simulink model "test_cosim_hydraulics"  (Simulink 7.4)
settings: Solver=ode15s  StartTime=0.0  StopTime=20.0  MaxStep=0.2  RelTol=1e-3
InitFcn:
  | valve_orifice_area = 0.16;
  | x0 = 0.8;
undefined symbols (not defined in the file): CEcosimulation, CoSimulate1, sigbuilder_block
libraries: fl_lib x21, sh_lib x10, nesl_utility x9, instrumentlib x2
Description:
  | Power-Assisted Steering Mechanism
  | 
  | The model represents a simplified version of a power-assisted steering mechanism
  | showing all its major parts: double-acting hydraulic cylinder; rotational valve; fixed-
  | displacement pump;  pressure-relief valve; mechanical load consisting of a reduced
  | to a driving shaft inertia, damping, and stiffness; and torsion bar installed between the
  | steering wheel and the pinion of a rack-and-pinion mechanism.
  | The rotation of the steering wheel causes the torsion bar to twist with respect to the
  | pinion position. The deformation of the bar is transformed into opening of the rotational
  | valve, which connects ports of the cylinder to pressure or exhaust lines depending on
  | the direction of rotation. If deformation exceeds 9 deg the wheel is connected directly
  | to the pinion through the hard stops installed in parallel with the torsion bar.
  | The cylinder moves the steering rods and, at the same time, twists the torsion rod
  | in the opposite direction until the valve is in neutral position.
  | 
  | 
  | Copyright 2008-2009 The MathWorks(TM), Inc.
settings Model: Creator=vtchkalo  LastModifiedBy=tasora  ExtModeAutoUpdateStatusClock=off
settings SolverCC: InitialStep=1e-6
settings OptimizationCC: InitFltsAndDblsToZero=on
settings DebuggingCC: SaveWithParameterizedLinksMsg=none  SignalResolutionControl=TryResolveAllWithWarning  SolverPrmCheckMsg=none
settings GRTTargetCC: TargetFcnLib=ansi_tfl_tmw.mat

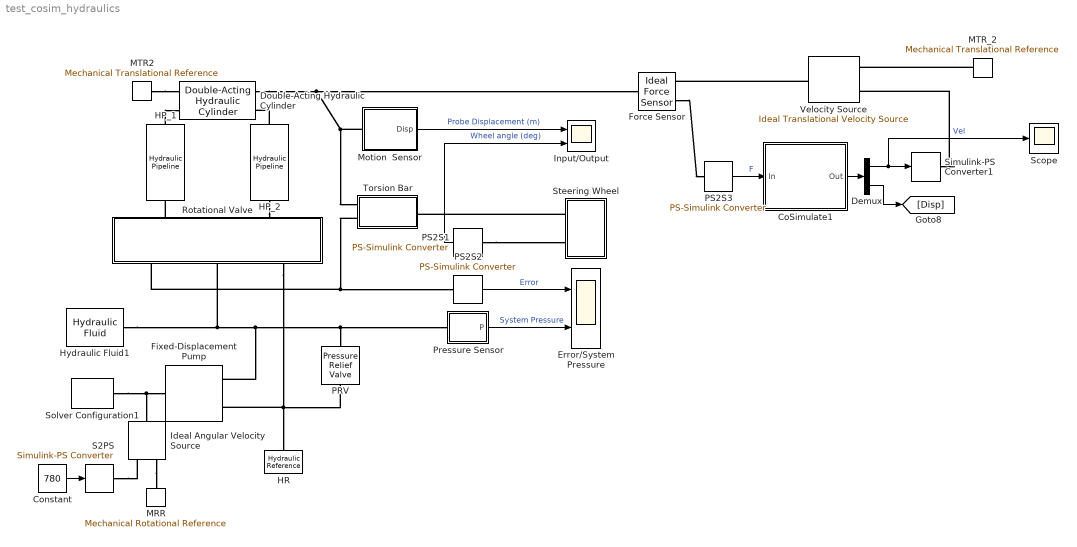
== system test_cosim_hydraulics ==
  CoSimulate1 : Subsystem  Description=|  Priority=100  AncestorBlock=CEcosimulation/CoSimulate1  mask{com_step=0.001, tcp_data_size=2, host_name=localhost, tcp_port=50009, tcp_timeout=15}
      | This block can be used to exchange data with Chrono::Engine.                                                                                      
      | A Chrono::Engine program with a running ChCosimulation inferface must be started, it will work as a server; then the Simulink program must be run.
      | Note! check that the dimensions of the exchanged vectors do match!
      mask prompts: com_step "Communication step size"; tcp_data_size "N. of scalars received from C::E (as block output)"; host_name "TCP host name (ex. 'localhost', or 'www.myhost.com')"; tcp_port "TCP port (ex. 50007)"; tcp_timeout "TCP timeout (seconds)"
      mask init:
      | block_receive = [gcb, '/TCP Receive'];
      | set_param(block_receive, 'SampleTime', num2str(com_step));
      | set_param(block_receive, 'Host', host_name);
      | set_param(block_receive, 'Port', num2str(tcp_port));
      | set_param(block_receive, 'DataSize', num2str(tcp_data_size+1));
      | set_param(block_receive, 'Timeout', num2str(tcp_timeout));
      | block_send = [gcb, '/TCP Send'];
      | set_param(block_send, 'Host', host_name);
      | set_param(block_send, 'Port', num2str(tcp_port));
      mask Display:
      | image(imread('block_logo.png'))
      | disp('C::E                   ')
  Constant : Constant  Value=780  OutDataType=sfix(16)  OutScaling=2^0
  Demux : Demux  Outputs=2
  Double-Acting Hydraulic Cylinder : sh_lib/Hydraulic Cylinders/Double-Acting Hydraulic Cylinder  Tag=Factory Generic  DialogController=NetworkEngine.DynNeDlgSource  SystemSampleTime=-1  area_A=9.1 cm^2  area_B=9.1 cm^2  stroke=18.4 cm  init_pos=9.2 cm  dead_vol_A=1e-04 m^3  dead_vol_B=1e-04 m^3  k_sh=1.4  stiff=1e+06 N/m  D=150 N/(m/s)  or=1  LocalVarLogging=[]
  Error/System Pressure : Scope  NumInputPorts=2
      settings: TimeRange=20  YMin=-0.4~7  YMax=0.4~10  SaveName=ScopeDataCE
  Fixed-Displacement Pump : sh_lib/Pumps and Motors/Fixed-Displacement Pump  Tag=Factory Generic  DialogController=NetworkEngine.DynNeDlgSource  SystemSampleTime=-1  D=1.14e-06 m^3/rad  efficiency_vol=0.92  efficiency_tot=0.8  pr_nominal=1e+07 Pa  w_nominal=188 rad/s  visc_nominal=18 cSt  pump_delivery_Log=off  leakage_flow_Log=off  torque_Log=off  power_hyd_Log=off  pressure_diff_Log=off  shaft_ang_vel_Log=off  LocalVarNames=|pump_delivery|leakage_flow|torque|power_hyd|pressure_diff|shaft_ang_vel  LocalVarDescs=|Pump delivery (m^3/s)|Leakage flow rate (m^3/s)|Driving shaft torque (N*m)|Output flow power (W)|Pressure differential (Pa)|Driving shaft angular velocity (rad/s)  LocalVarLogging=[0 0 0 0 0 0]
  Force Sensor : fl_lib/Mechanical/Mechanical Sensors/Ideal Force Sensor  Tag=Factory Generic  DialogController=NetworkEngine.DynNeDlgSource  SystemSampleTime=-1  v_Log=off  f_Log=off  LocalVarNames=|v|f  LocalVarDescs=|v|f  LocalVarLogging=[]
  HP_1 : sh_lib/Pipelines/Hydraulic Pipeline  Tag=Factory Generic  DialogController=NetworkEngine.DynNeDlgSource  SystemSampleTime=-1  cs_type=1  d_in=6 mm  area=1e-04 m^2  D_h=0.0112 m  s_factor=64  length=1.8 m  length_ad=1 m  roughness=1.5e-05 m  Re_lam=2e+03  Re_turb=4e+03  wall_type=1  pr_r_coef=2e-12 m/Pa  time_const=0.01 s  k_sh=1.4  LocalVarLogging=[]
  HP_2 : sh_lib/Pipelines/Hydraulic Pipeline  Tag=Factory Generic  DialogController=NetworkEngine.DynNeDlgSource  SystemSampleTime=-1  cs_type=1  d_in=6 mm  area=1e-04 m^2  D_h=0.0112 m  s_factor=64  length=1.6 m  length_ad=1 m  roughness=1.5e-05 m  Re_lam=2e+03  Re_turb=4e+03  wall_type=1  pr_r_coef=2e-12 m/Pa  time_const=0.01 s  k_sh=1.4  LocalVarLogging=[]
  HR : fl_lib/Hydraulic/Hydraulic Elements/Hydraulic Reference  Tag=Factory Generic  DialogController=NetworkEngine.DynNeDlgSource  SystemSampleTime=-1  q_Log=off  LocalVarNames=|q  LocalVarDescs=|q  LocalVarLogging=[]
  Hydraulic Fluid1 : sh_lib/Hydraulic Utilities/Hydraulic Fluid  Tag=Factory Generic  DialogController=NetworkEngine.DynNeDlgSource  SystemSampleTime=-1  DataSource=1  SelFluid=9  SysTemp=60 c  TrapAir=0.005  ViscDerFactor=1  LocalVarLogging=[]
  Ideal Angular Velocity Source : fl_lib/Mechanical/Mechanical Sources/Ideal Angular Velocity Source  Tag=Factory Generic  DialogController=NetworkEngine.DynNeDlgSource  SystemSampleTime=-1  w_Log=off  t_Log=off  LocalVarNames=|torque|rel_velocity|power  LocalVarDescs=|Torque (N*m)|Relative velocity (rad/s)|Power generated by the sourcec(W)  LocalVarLogging=[0 0 0]
  Input/Output : Scope  NumInputPorts=2
      settings: TimeRange=20  YMin=-0.001~0  YMax=0.009~15
  MRR : fl_lib/Mechanical/Rotational Elements/Mechanical Rotational Reference  Tag=Factory Generic  DialogController=NetworkEngine.DynNeDlgSource  SystemSampleTime=-1  t_Log=off  LocalVarNames=|t  LocalVarDescs=|t  LocalVarLogging=[]
  MTR2 : fl_lib/Mechanical/Translational Elements/Mechanical Translational Reference  Tag=Factory Generic  DialogController=NetworkEngine.DynNeDlgSource  SystemSampleTime=-1  f_Log=off  LocalVarNames=|f  LocalVarDescs=|f  LocalVarLogging=[]
  MTR_2 : fl_lib/Mechanical/Translational Elements/Mechanical Translational Reference  Tag=Factory Generic  DialogController=NetworkEngine.DynNeDlgSource  SystemSampleTime=-1  f_Log=off  LocalVarNames=|f  LocalVarDescs=|f  LocalVarLogging=[]
  Motion  Sensor : Subsystem
  PRV : sh_lib/Valves/Pressure Control Valves/Pressure Relief Valve  Tag=Factory Generic  DialogController=NetworkEngine.DynNeDlgSource  SystemSampleTime=-1  area_max=0.46 cm^2  pres_set=12 bar  reg_range=2.1 bar  C_d=0.7  Re_cr=12  A_leak=1e-9 m^2  flow_rate_Log=off  pr_drop_Log=off  power_Log=off  area_Log=off  Re_Log=off  LocalVarNames=|flow_rate|pr_drop|power|area|Re  LocalVarDescs=|Flow rate through the valve (m^3/s)|Pressure differential across the valve (Pa)|Hydraulic loss power (W)|Instantaneous passage area (m^2)|Reynolds number  LocalVarLogging=[0 0 0 0 0]
  PS2S1 : nesl_utility/PS-Simulink Converter  DialogController=NetworkEngine.DynNeUtilDlgSource  SystemSampleTime=-1  PhysicalDomain=network_engine_domain  LeftPortType=input  RightPortType=output  SubClassName=ps_output  Unit=deg  AffineConversion=off
  PS2S2 : nesl_utility/PS-Simulink Converter  DialogController=NetworkEngine.DynNeUtilDlgSource  SystemSampleTime=-1  PhysicalDomain=network_engine_domain  LeftPortType=input  RightPortType=output  SubClassName=ps_output  Unit=deg  AffineConversion=off
  PS2S3 : nesl_utility/PS-Simulink Converter  DialogController=NetworkEngine.DynNeUtilDlgSource  SystemSampleTime=-1  PhysicalDomain=network_engine_domain  LeftPortType=input  RightPortType=output  SubClassName=ps_output  Unit=N  AffineConversion=off
  Pressure Sensor : Subsystem
  Rotational Valve : Subsystem
  S2PS : nesl_utility/Simulink-PS Converter  DialogController=NetworkEngine.DynNeUtilDlgSource  SystemSampleTime=-1  PhysicalDomain=network_engine_domain  LeftPortType=input  RightPortType=output  SubClassName=ps_input  Unit=rpm  AffineConversion=off  InputFilterTimeConstant=.001  UdotUserProvided=0
  Scope : Scope
  Simulink-PS Converter1 : nesl_utility/Simulink-PS Converter  DialogController=NetworkEngine.DynNeUtilDlgSource  SystemSampleTime=-1  PhysicalDomain=network_engine_domain  LeftPortType=input  RightPortType=output  SubClassName=ps_input  Unit=1  AffineConversion=off  InputFilterTimeConstant=.001  UdotUserProvided=0
  Solver Configuration1 : nesl_utility/Solver Configuration  DialogController=NetworkEngine.DynNeUtilDlgSource  SystemSampleTime=-1  PhysicalDomain=network_engine_domain  LeftPortType=input  RightPortType=generic  SubClassName=solver  Accelerate=off  Profile=off  Reg=off  Der=off  ResidualTolerance=1e-9  MaxNonlinIter=12  MaxModeIter=2  DoFixedCost=off  DoDC=off  LinearAlgebra=Sparse  LocalSolverSampleTime=.001  LocalSolverChoice=NE_BACKWARD_EULER_ADVANCER  UseLocalSolver=off
  Steering Wheel : Subsystem
  Torsion Bar : Subsystem
  Velocity Source : fl_lib/Mechanical/Mechanical Sources/Ideal Translational Velocity Source  DialogController=NetworkEngine.DynNeDlgSource  SystemSampleTime=-1  v_Log=off  f_Log=off  LocalVarNames=|v|f  LocalVarDescs=|v|f  LocalVarLogging=[0 0]
  wires:
  Constant/1 -> S2PS/1
  Motion  Sensor/1(Disp) -> Input/Output/1  "Probe Displacement (m)"
  PS2S1/1 -> Input/Output/2  "Wheel angle (deg)"
  PS2S2/1 -> Error/System Pressure/1  "Error"
  Pressure Sensor/1(P) -> Error/System Pressure/2  "System Pressure"
  PS2S3/1 -> CoSimulate1/1(In)  "F"
  CoSimulate1/1(Out) -> Demux/1
  Demux/1 -> Simulink-PS Converter1/1, Scope/1  "Vel"
  Demux/2 -> [Disp]
  connections:
  Double-Acting Hydraulic Cylinder/RConn1 -- Torsion Bar/RConn1 -- Motion  Sensor/LConn1 -- Force Sensor/LConn1
  HP_2/RConn1 -- Rotational Valve/RConn2
  Steering Wheel/RConn1 -- Torsion Bar/LConn1
  Rotational Valve/RConn1 -- HP_1/LConn1
  HP_1/RConn1 -- Double-Acting Hydraulic Cylinder/LConn2
  Ideal Angular Velocity Source/RConn2 -- MRR/LConn1
  MTR2/LConn1 -- Double-Acting Hydraulic Cylinder/LConn1
  HP_2/LConn1 -- Double-Acting Hydraulic Cylinder/RConn2
  S2PS/RConn1 -- Ideal Angular Velocity Source/RConn1
  Solver Configuration1/RConn1 -- Fixed-Displacement Pump/LConn1 -- Ideal Angular Velocity Source/LConn1
  PS2S1/LConn1 -- Steering Wheel/RConn2
  Torsion Bar/RConn2 -- PS2S2/LConn1 -- Rotational Valve/LConn1
  Hydraulic Fluid1/RConn1 -- Rotational Valve/LConn2 -- Fixed-Displacement Pump/RConn1 -- Pressure Sensor/LConn1 -- PRV/LConn1
  Rotational Valve/LConn3 -- Fixed-Displacement Pump/RConn2 -- HR/LConn1 -- PRV/RConn1
  Velocity Source/LConn1 -- Force Sensor/RConn1
  Force Sensor/RConn2 -- PS2S3/LConn1
  Simulink-PS Converter1/RConn1 -- Velocity Source/RConn1
  MTR_2/LConn1 -- Velocity Source/RConn2

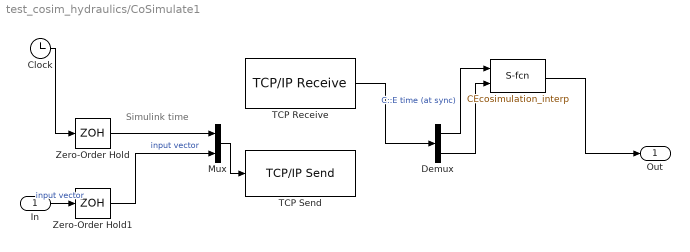
== system test_cosim_hydraulics/CoSimulate1 ==
  note: Simulink time
  In : Inport
  " " : M-S-Function  FunctionName=CEcosimulation_interp
  Clock : Clock
      settings: Decimation=10
  Demux : Demux  Outputs=[1 -1]
  Mux : Mux  Inputs=2
  TCP Receive : instrumentlib/TCP//IP Receive  Priority=1  DialogController=instrumentcreatedialog  DialogControllerArgs=DataTag0  Host=localhost  Port=50009  DataSize=3  EnableBlockingMode=on  Timeout=15  SampleTime=0.001  DataType=double  ByteOrder=LittleEndian
  TCP Send : instrumentlib/TCP//IP Send  Priority=2  DialogController=instrumentcreatedialog  DialogControllerArgs=DataTag1  Host=localhost  Port=50009  EnableBlockingMode=on  Timeout=10  ByteOrder=LittleEndian
  Zero-Order Hold : ZeroOrderHold  Priority=0  SampleTime=com_step
  Zero-Order Hold1 : ZeroOrderHold  Priority=0  SampleTime=com_step
  Out : Outport
  wires:
  " "/1 -> Out/1
  Demux/2 -> " "/2
  Demux/1 -> " "/1  "C::E time (at sync)"
  Zero-Order Hold/1 -> Mux/1
  Zero-Order Hold1/1 -> Mux/2  "input vector"
  Mux/1 -> TCP Send/1
  Clock/1 -> Zero-Order Hold/1
  In/1 -> Zero-Order Hold1/1  "input vector"
  TCP Receive/1 -> Demux/1

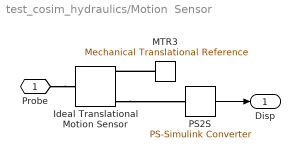
== system test_cosim_hydraulics/Motion  Sensor ==
  Ideal Translational Motion Sensor : fl_lib/Mechanical/Mechanical Sensors/Ideal Translational Motion Sensor  Tag=Factory Generic  DialogController=NetworkEngine.DynNeDlgSource  SystemSampleTime=-1  offset=0 m  v_Log=off  f_Log=off  x_Log=off  LocalVarNames=|v|f|x  LocalVarDescs=|v|f|x  LocalVarLogging=[]
  MTR3 : fl_lib/Mechanical/Translational Elements/Mechanical Translational Reference  Tag=Factory Generic  DialogController=NetworkEngine.DynNeDlgSource  SystemSampleTime=-1  f_Log=off  LocalVarNames=|f  LocalVarDescs=|f  LocalVarLogging=[]
  PS2S : nesl_utility/PS-Simulink Converter  DialogController=NetworkEngine.DynNeUtilDlgSource  SystemSampleTime=-1  PhysicalDomain=network_engine_domain  LeftPortType=input  RightPortType=output  SubClassName=ps_output  Unit=1  AffineConversion=off
  Probe : PMIOPort  Port=1  Side=Left
  Disp : Outport  OutDataType=sfix(16)  OutScaling=2^0
  wires:
  PS2S/1 -> Disp/1
  connections:
  Probe/RConn1 -- Ideal Translational Motion Sensor/LConn1
  Ideal Translational Motion Sensor/RConn3 -- PS2S/LConn1
  MTR3/LConn1 -- Ideal Translational Motion Sensor/RConn1

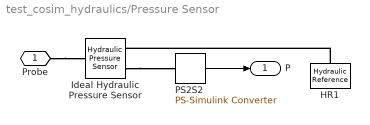
== system test_cosim_hydraulics/Pressure Sensor ==
  HR1 : fl_lib/Hydraulic/Hydraulic Elements/Hydraulic Reference  Tag=Factory Generic  DialogController=NetworkEngine.DynNeDlgSource  SystemSampleTime=-1  q_Log=off  LocalVarNames=|q  LocalVarDescs=|q  LocalVarLogging=[]
  Ideal Hydraulic Pressure Sensor : fl_lib/Hydraulic/Hydraulic Sensors/Hydraulic Pressure Sensor  Tag=Factory Generic  DialogController=NetworkEngine.DynNeDlgSource  SystemSampleTime=-1  q_Log=off  p_Log=off  LocalVarNames=|q|p  LocalVarDescs=|q|p  LocalVarLogging=[]
  PS2S2 : nesl_utility/PS-Simulink Converter  DialogController=NetworkEngine.DynNeUtilDlgSource  SystemSampleTime=-1  PhysicalDomain=network_engine_domain  LeftPortType=input  RightPortType=output  SubClassName=ps_output  Unit=bar  AffineConversion=off
  Probe : PMIOPort  Port=1  Side=Left
  P : Outport  OutDataType=sfix(16)  OutScaling=2^0
  wires:
  PS2S2/1 -> P/1
  connections:
  Probe/RConn1 -- Ideal Hydraulic Pressure Sensor/LConn1
  Ideal Hydraulic Pressure Sensor/RConn2 -- PS2S2/LConn1
  HR1/LConn1 -- Ideal Hydraulic Pressure Sensor/RConn1

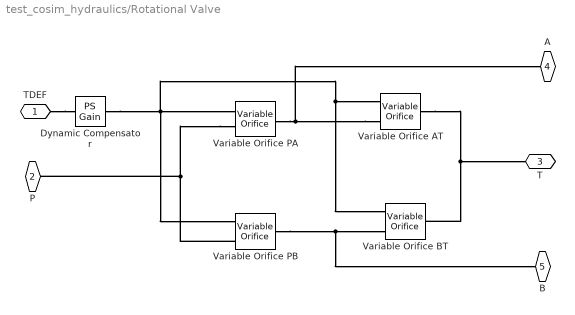
== system test_cosim_hydraulics/Rotational Valve ==
  Dynamic Compensator : fl_lib/Physical Signals/Functions/PS Gain  Tag=Factory Generic  DialogController=NetworkEngine.DynNeDlgSource  SystemSampleTime=-1  gain=0.0212  LocalVarLogging=[]
  Variable Orifice AT : sh_lib/Orifices/Variable Orifice  Tag=Factory Generic  DialogController=NetworkEngine.DynNeDlgSource  SystemSampleTime=-1  mdl_type=1  area_max=valve_orifice_area cm^2  opening_max=6 mm  opening_tab="[  -0.002 0 0.005 0.015 ] m"  area_tab="[  1e-12 4e-12 1e-05 1.02e-05 ] m^2"  pressure_tab="[  -5e+06 -2e+06 2e+06 5e+06 ] Pa"  flow_rate_tab="[  -1e-12 -6e-14 6e+12 1e+11 ; -8e-08 -4e-08 4e+06 8e+06 ; -0.0025 -0.00103 0.001 0.0024 ; -0.00258 -0.001032 0.00106 0.00247 ; ] m^3/s"  interp_method=1  extrap_method=1  or=1  C_d=0.7  x_0=x0 mm  Re_cr=12  A_leak=1e-12 m^2  flow_rate_Log=off  pr_drop_Log=off  Re_Log=off  orif_opening_Log=off  power_Log=off  LocalVarNames=|flow_rate|pr_drop|Re|orif_opening|power  LocalVarDescs=|Flow rate through the orifice (m^3)|Pressure drop across the orifice (Pa)|Reynolds number|Orifice opening (m)|Power dissipated in the orifice (W)  LocalVarLogging=[0 0 0 0 0]
  Variable Orifice BT : sh_lib/Orifices/Variable Orifice  Tag=Factory Generic  DialogController=NetworkEngine.DynNeDlgSource  SystemSampleTime=-1  mdl_type=1  area_max=valve_orifice_area cm^2  opening_max=6 mm  opening_tab="[  -0.002 0 0.005 0.015 ] m"  area_tab="[  1e-12 4e-12 1e-05 1.02e-05 ] m^2"  pressure_tab="[  -5e+06 -2e+06 2e+06 5e+06 ] Pa"  flow_rate_tab="[  -1e-12 -6e-14 6e+12 1e+11 ; -8e-08 -4e-08 4e+06 8e+06 ; -0.0025 -0.00103 0.001 0.0024 ; -0.00258 -0.001032 0.00106 0.00247 ; ] m^3/s"  interp_method=1  extrap_method=1  or=1  C_d=0.7  x_0=x0 mm  Re_cr=12  A_leak=1e-12 m^2  flow_rate_Log=off  pr_drop_Log=off  Re_Log=off  orif_opening_Log=off  power_Log=off  LocalVarNames=|flow_rate|pr_drop|Re|orif_opening|power  LocalVarDescs=|Flow rate through the orifice (m^3)|Pressure drop across the orifice (Pa)|Reynolds number|Orifice opening (m)|Power dissipated in the orifice (W)  LocalVarLogging=[0 0 0 0 0]
  Variable Orifice PA : sh_lib/Orifices/Variable Orifice  Tag=Factory Generic  DialogController=NetworkEngine.DynNeDlgSource  SystemSampleTime=-1  mdl_type=1  area_max=valve_orifice_area cm^2  opening_max=6 mm  opening_tab="[  -0.002 0 0.005 0.015 ] m"  area_tab="[  1e-12 4e-12 1e-05 1.02e-05 ] m^2"  pressure_tab="[  -5e+06 -2e+06 2e+06 5e+06 ] Pa"  flow_rate_tab="[  -1e-12 -6e-14 6e+12 1e+11 ; -8e-08 -4e-08 4e+06 8e+06 ; -0.0025 -0.00103 0.001 0.0024 ; -0.00258 -0.001032 0.00106 0.00247 ; ] m^3/s"  interp_method=1  extrap_method=1  or=1  C_d=0.7  x_0=x0 mm  Re_cr=12  A_leak=1e-12 m^2  flow_rate_Log=off  pr_drop_Log=off  Re_Log=off  orif_opening_Log=off  power_Log=off  LocalVarNames=|flow_rate|pr_drop|Re|orif_opening|power  LocalVarDescs=|Flow rate through the orifice (m^3)|Pressure drop across the orifice (Pa)|Reynolds number|Orifice opening (m)|Power dissipated in the orifice (W)  LocalVarLogging=[0 0 0 0 0]
  Variable Orifice PB : sh_lib/Orifices/Variable Orifice  Tag=Factory Generic  DialogController=NetworkEngine.DynNeDlgSource  SystemSampleTime=-1  mdl_type=1  area_max=valve_orifice_area cm^2  opening_max=6 mm  opening_tab="[  -0.002 0 0.005 0.015 ] m"  area_tab="[  1e-12 4e-12 1e-05 1.02e-05 ] m^2"  pressure_tab="[  -5e+06 -2e+06 2e+06 5e+06 ] Pa"  flow_rate_tab="[  -1e-12 -6e-14 6e+12 1e+11 ; -8e-08 -4e-08 4e+06 8e+06 ; -0.0025 -0.00103 0.001 0.0024 ; -0.00258 -0.001032 0.00106 0.00247 ; ] m^3/s"  interp_method=1  extrap_method=1  or=2  C_d=0.7  x_0=x0 mm  Re_cr=12  A_leak=1e-12 m^2  flow_rate_Log=off  pr_drop_Log=off  Re_Log=off  orif_opening_Log=off  power_Log=off  LocalVarNames=|flow_rate|pr_drop|Re|orif_opening|power  LocalVarDescs=|Flow rate through the orifice (m^3)|Pressure drop across the orifice (Pa)|Reynolds number|Orifice opening (m)|Power dissipated in the orifice (W)  LocalVarLogging=[0 0 0 0 0]
  TDEF : PMIOPort  Port=1  Side=Left
  P : PMIOPort  Port=2  Side=Left
  T : PMIOPort  Port=3  Side=Left
  A : PMIOPort  Port=4  Side=Right
  B : PMIOPort  Port=5  Side=Right
  connections:
  Dynamic Compensator/RConn1 -- Variable Orifice PA/LConn1 -- Variable Orifice PB/LConn1 -- Variable Orifice AT/LConn1 -- Variable Orifice BT/LConn1
  Variable Orifice AT/LConn2 -- A/RConn1 -- Variable Orifice PA/RConn1
  Variable Orifice AT/RConn1 -- T/RConn1 -- Variable Orifice BT/RConn1
  Variable Orifice PB/RConn1 -- Variable Orifice BT/LConn2 -- B/RConn1
  Variable Orifice PA/LConn2 -- P/RConn1 -- Variable Orifice PB/LConn2
  TDEF/RConn1 -- Dynamic Compensator/LConn1

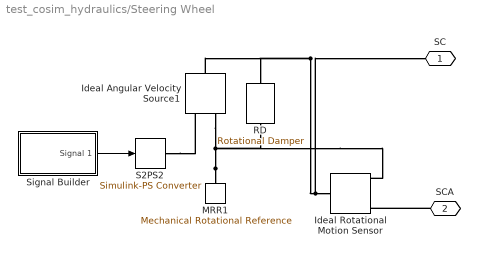
== system test_cosim_hydraulics/Steering Wheel ==
  Ideal Angular Velocity Source1 : fl_lib/Mechanical/Mechanical Sources/Ideal Angular Velocity Source  Tag=Factory Generic  DialogController=NetworkEngine.DynNeDlgSource  SystemSampleTime=-1  w_Log=off  t_Log=off  LocalVarNames=|torque|rel_velocity|power  LocalVarDescs=|Torque (N*m)|Relative velocity (rad/s)|Power generated by the sourcec(W)  LocalVarLogging=[0 0 0]
  Ideal Rotational Motion Sensor : fl_lib/Mechanical/Mechanical Sensors/Ideal Rotational Motion Sensor  Tag=Factory Generic  DialogController=NetworkEngine.DynNeDlgSource  SystemSampleTime=-1  offset=0 rad  w_Log=off  t_Log=off  phi_Log=off  LocalVarNames=|w|t|phi  LocalVarDescs=|w|t|phi  LocalVarLogging=[]
  MRR1 : fl_lib/Mechanical/Rotational Elements/Mechanical Rotational Reference  Tag=Factory Generic  DialogController=NetworkEngine.DynNeDlgSource  SystemSampleTime=-1  t_Log=off  LocalVarNames=|t  LocalVarDescs=|t  LocalVarLogging=[]
  RD : fl_lib/Mechanical/Rotational Elements/Rotational Damper  Tag=Factory Generic  DialogController=NetworkEngine.DynNeDlgSource  SystemSampleTime=-1  D=0.001 N*m/(rad/s)  t_Log=off  w_Log=off  LocalVarNames=|torque|velocity|power  LocalVarDescs=|Damping torque (N*m)|Damper relative velocity (rad/s)|Power dissipated in the damper (W)  LocalVarLogging=[0 0 0]
  S2PS2 : nesl_utility/Simulink-PS Converter  DialogController=NetworkEngine.DynNeUtilDlgSource  SystemSampleTime=-1  PhysicalDomain=network_engine_domain  LeftPortType=input  RightPortType=output  SubClassName=ps_input  Unit=rpm  AffineConversion=off  InputFilterTimeConstant=.001  UdotUserProvided=0
  Signal Builder : Subsystem  Tag=STV Subsys  LoadFcn=sigbuilder_block('load');  StartFcn=sigbuilder_block('start');  StopFcn=sigbuilder_block('stop');  ClipboardFcn=sigbuilder_block('clipboard');  mask(Sigbuilder block){}
      mask help: Sigbuilder GUI
      mask init:
      | if ~strcmp(get_param(bdroot(gcbh),'SimulationStatus'),'stopped') tuvar = sigbuilder_block('maskInit'); end
      settings: CopyFcn=sigbuilder_block('copy');  DeleteFcn=sigbuilder_block('delete');  ModelCloseFcn=sigbuilder_block('modelClose');  PreSaveFcn=sigbuilder_block('preSave');  NameChangeFcn=sigbuilder_block('namechange');  OpenFcn=sigbuilder_block('open',[437.6 199.2 550.4 400 ]);  CloseFcn=sigbuilder_block('close');
      mask Display: plot(0,0,100,100,[10,10,40,40,10],[80,20,20,80,80],[40,10],[50,50], [40,27,10],[65,72,56],[40,25,25,10],[28,28,43,43]);
  SC : PMIOPort  Port=1  Side=Right
  SCA : PMIOPort  Port=2  Side=Right
  wires:
  Signal Builder/1(Signal 1) -> S2PS2/1
  connections:
  SCA/RConn1 -- Ideal Rotational Motion Sensor/RConn3
  MRR1/LConn1 -- Ideal Angular Velocity Source1/RConn2 -- RD/RConn1 -- Ideal Rotational Motion Sensor/RConn1
  S2PS2/RConn1 -- Ideal Angular Velocity Source1/RConn1
  Ideal Rotational Motion Sensor/LConn1 -- SC/RConn1 -- RD/LConn1 -- Ideal Angular Velocity Source1/LConn1

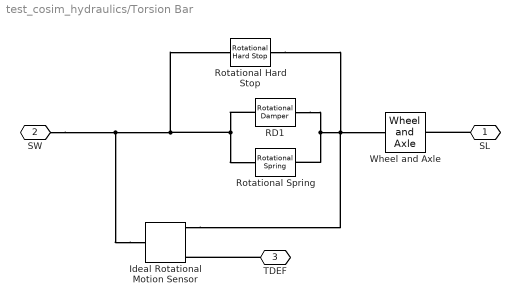
== system test_cosim_hydraulics/Torsion Bar ==
  Ideal Rotational Motion Sensor : fl_lib/Mechanical/Mechanical Sensors/Ideal Rotational Motion Sensor  Tag=Factory Generic  DialogController=NetworkEngine.DynNeDlgSource  SystemSampleTime=-1  offset=0 rad  w_Log=off  t_Log=off  phi_Log=off  LocalVarNames=|w|t|phi  LocalVarDescs=|w|t|phi  LocalVarLogging=[]
  RD1 : fl_lib/Mechanical/Rotational Elements/Rotational Damper  Tag=Factory Generic  DialogController=NetworkEngine.DynNeDlgSource  SystemSampleTime=-1  D=0.01 N*m/(rad/s)  t_Log=off  w_Log=off  LocalVarNames=|torque|velocity|power  LocalVarDescs=|Damping torque (N*m)|Damper relative velocity (rad/s)|Power dissipated in the damper (W)  LocalVarLogging=[0 0 0]
  Rotational Hard Stop : fl_lib/Mechanical/Rotational Elements/Rotational Hard Stop  Tag=Factory Generic  DialogController=NetworkEngine.DynNeDlgSource  SystemSampleTime=-1  upper_bnd=9 deg  lower_bnd=-9 deg  stiff_up=1e+06 N*m/rad  stiff_low=1e+06 N*m/rad  D_up=0.01 N*m/(rad/s)  D_low=0.01 N*m/(rad/s)  t_Log=off  w_Log=off  phi_Log=off  LocalVarNames=|contact_torque|rel_angle  LocalVarDescs=|Contact torque (N*m)|Slider-case relative angle (rad)  LocalVarLogging=[0 0]
  Rotational Spring : fl_lib/Mechanical/Rotational Elements/Rotational Spring  Tag=Factory Generic  DialogController=NetworkEngine.DynNeDlgSource  SystemSampleTime=-1  spr_rate=10 N*m/rad  init_def=0 rad  t_Log=off  w_Log=off  phi_Log=off  LocalVarNames=|torque|deformation  LocalVarDescs=|Spring torque (N*m)|Spring deformation (rad)  LocalVarLogging=[0 0]
  Wheel and Axle : fl_lib/Mechanical/Mechanisms/Wheel and Axle  Tag=Factory Generic  DialogController=NetworkEngine.DynNeDlgSource  SystemSampleTime=-1  R=3.8 cm  or=1  torque_A_Log=off  force_P_Log=off  ang_velocity_Log=off  velocity_Log=off  LocalVarNames=|torque_A|force_P|ang_velocity|velocity  LocalVarDescs=|Axle torque (N*m)|Periphery force (N)|Axle angular velocity (rad/s)|Periphery velocity (m/s)  LocalVarLogging=[0 0 0 0]
  SL : PMIOPort  Port=1  Side=Right
  SW : PMIOPort  Port=2  Side=Left
  TDEF : PMIOPort  Port=3  Side=Right
  connections:
  TDEF/RConn1 -- Ideal Rotational Motion Sensor/RConn3
  SL/RConn1 -- Wheel and Axle/RConn1
  Rotational Hard Stop/RConn1 -- Wheel and Axle/LConn1 -- Rotational Spring/RConn1 -- RD1/RConn1 -- Ideal Rotational Motion Sensor/RConn1
  Ideal Rotational Motion Sensor/LConn1 -- Rotational Hard Stop/LConn1 -- Rotational Spring/LConn1 -- RD1/LConn1 -- SW/RConn1

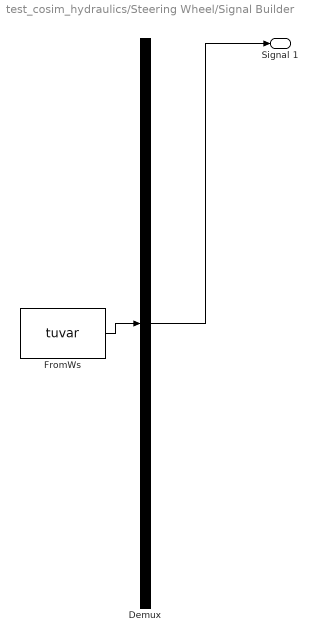
== system test_cosim_hydraulics/Steering Wheel/Signal Builder ==
  Demux : Demux  Tag=STV Demux  Outputs=1
  FromWs : FromWorkspace  Tag=STV FromWs  VariableName=tuvar  SampleTime=0  SigBuilderData=DataTag2  VnvData=DataTag3
      SigBuilderData=|
      | channels.label = 'Signal 1'
      | channels.allXData = {[0 1.96 2.4 4.05 4.5 5.95 6.75 8.05 8.4 10 10.35 11.7 12 13.85 14.2 15.7 15.95 20]}
      | channels.allYData = {[0 0 0.99 1 0 0 -1 -1 0 0 -1 -0.99 0 0 1 1 0 0]}
      | common.afterFinalStr = 'Extrapolate'
      | common.sampleTime = 0
      | dataSet.timeRange = [0 20]
      | dataSet.name = 'Group 1'
  Signal 1 : Outport  Tag=STV Outport  OutDataType=sfix(16)  OutScaling=2^0
  wires:
  FromWs/1 -> Demux/1
  Demux/1 -> Signal 1/1
